simulink model "EPSAC_SM_BOOST"  (R2016a)
settings: Solver=VariableStepAuto  StartTime=0.0  StopTime=5  RelTol=1e-3
libraries: powerlib x11
settings Model: Creator=jorda  LastModifiedBy=jorda

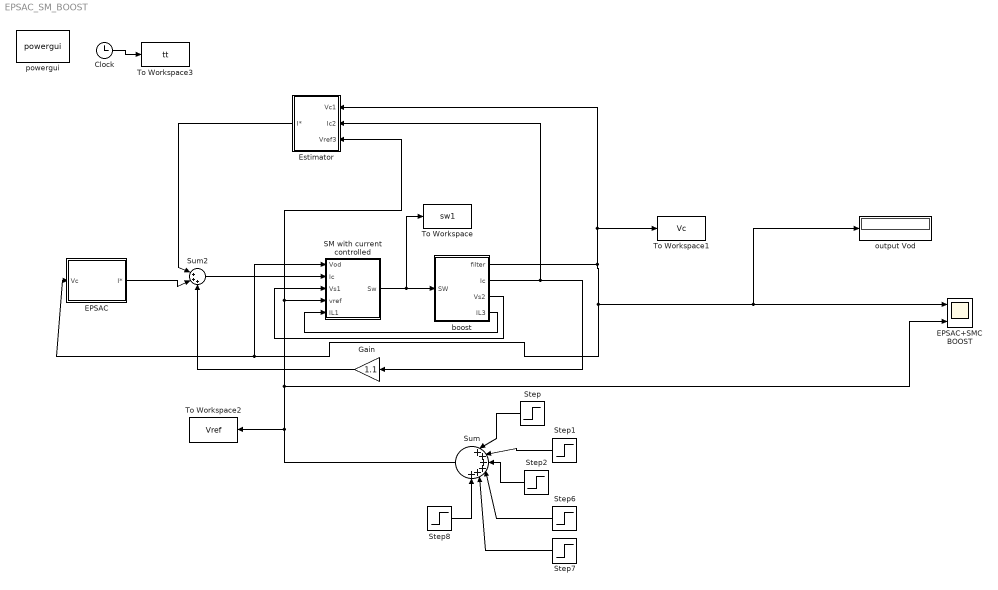
== system EPSAC_SM_BOOST ==
  Clock : Clock
  EPSAC : Subsystem
  EPSAC+SMC BOOST : Scope  NumInputPorts=2
  Estimator : Subsystem
  Gain : Gain  Gain=1.1
  SM with current controlled : Subsystem
  Step : Step  Time=0.5  Before=20  After=21  SampleTime=0
  Step1 : Step  SampleTime=0
  Step2 : Step  Time=1.5  After=-2  SampleTime=0
  Step6 : Step  Time=2  After=-1  SampleTime=0
  Step7 : Step  Time=2.5  After=-1  SampleTime=0
  Step8 : Step  Time=3  After=2  SampleTime=0
  Sum : Sum  Inputs=|++++++
  Sum2 : Sum  Inputs=|+++
  To Workspace : ToWorkspace  VariableName=sw1  SampleTime=1e-3
  To Workspace1 : ToWorkspace  VariableName=Vc  SampleTime=1e-3
  To Workspace2 : ToWorkspace  VariableName=Vref  SampleTime=1e-3
  To Workspace3 : ToWorkspace  VariableName=tt  SampleTime=1e-3
  boost : Subsystem
  output Vod : Display
  powergui : powerlib/powergui  Priority=1  SimulationMode=Continuous  SolverType=Tustin/Backward Euler (TBE)  SampleTime=50e-6  frequency=60  SPID=off  DisableSnubberDevices=off  DisableRonSwitches=off  DisableVfSwitches=off  SwTol=0  DisplayEquations=off  Interpol=off  ExternalGateDelay=off  methode=off  Ts=10  FunctionMessages=off  echomessages=off  HookPort=off  EnableUseOfTLC=off  x0status=blocks  frequencyindice=0  Pbase=100e6  ErrMax=1e-4  Iterations=50  UnitsV=kV  UnitsW=MW  buscounter=0  RestoreLinks=warning  ResistiveCurrentMeasurement=off  Frange=[0:2:500]  Ylog=off  Xlog=on  ShowGrid=off  save=off  variable=ZData  structure=0  ZoomFFT=off  StartTime=0.0  cycles=1  DisplayStyle=1  fundamental=60  FreqAxis=off  MaxFrequency=1000  frequencyindicesteady=1  RmsSteady=1  display=off
  wires:
  boost/3(Vs2) -> SM with current controlled/3("Vs1 ")
  boost/1(filter) -> output Vod/1, EPSAC+SMC BOOST/1, SM with current controlled/1(Vod), EPSAC/1(Vc), Estimator/1(Vc1), To Workspace1/1
  SM with current controlled/1(Sw) -> To Workspace/1, boost/1(SW)
  boost/2(Ic) -> Estimator/2(Ic2), Gain/1
  Clock/1 -> To Workspace3/1
  Gain/1 -> Sum2/3
  Step/1 -> Sum/1
  Step1/1 -> Sum/2
  Step2/1 -> Sum/3
  Step6/1 -> Sum/4
  Step7/1 -> Sum/5
  Step8/1 -> Sum/6
  Sum/1 -> To Workspace2/1, EPSAC+SMC BOOST/2, Estimator/3(Vref3), SM with current controlled/4(vref)
  boost/4(IL3) -> SM with current controlled/5(IL1)
  Sum2/1 -> SM with current controlled/2(Ic)
  EPSAC/1(I*) -> Sum2/2
  Estimator/1(I*) -> Sum2/1

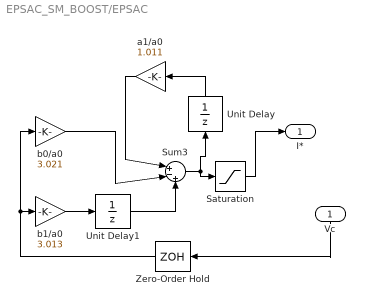
== system EPSAC_SM_BOOST/EPSAC ==
  Vc : Inport
  Saturation : Saturate  UpperLimit=0.4  LowerLimit=-0.4
  Sum3 : Sum  Inputs=|+-+
  Unit Delay : UnitDelay  SampleTime=1e-3
  Unit Delay1 : UnitDelay  SampleTime=1e-3
  Zero-Order Hold : ZeroOrderHold  SampleTime=1e-3
  a1/a0 : Gain  Gain=1.011
  b0/a0 : Gain  Gain=3.021
  b1/a0 : Gain  Gain=3.013
  I* : Outport
  wires:
  Vc/1 -> Zero-Order Hold/1
  Saturation/1 -> I*/1
  b0/a0/1 -> Sum3/2
  Zero-Order Hold/1 -> b0/a0/1, b1/a0/1
  b1/a0/1 -> Unit Delay1/1
  Unit Delay1/1 -> Sum3/3
  a1/a0/1 -> Sum3/1
  Unit Delay/1 -> a1/a0/1
  Sum3/1 -> Saturation/1, Unit Delay/1

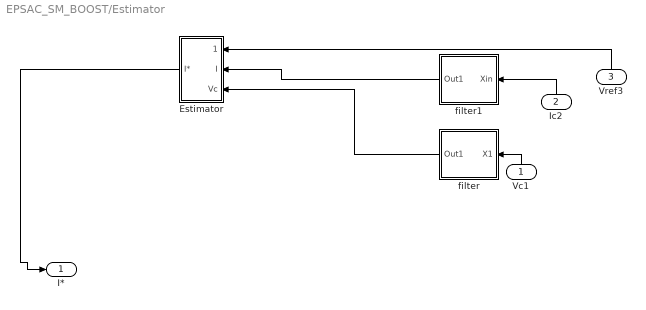
== system EPSAC_SM_BOOST/Estimator ==
  Vc1 : Inport
  Ic2 : Inport  Port=2
  Vref3 : Inport  Port=3
  Estimator : Subsystem
  filter : Subsystem
  filter1 : Subsystem
  I* : Outport
  wires:
  filter1/1(Out1) -> Estimator/2(I)
  Estimator/1(I*) -> I*/1
  Ic2/1 -> filter1/1(Xin)
  Vc1/1 -> filter/1(X1)
  Vref3/1 -> Estimator/1(Vref)
  filter/1(Out1) -> Estimator/3(Vc)

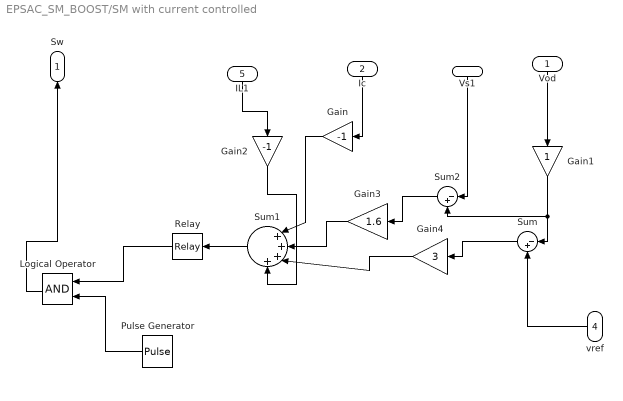
== system EPSAC_SM_BOOST/SM with current controlled ==
  Vod : Inport
  Ic : Inport  Port=2
  "Vs1 " : Inport  Port=3
  vref : Inport  Port=4
  IL1 : Inport  Port=5
  Gain : Gain  Gain=-1  ParamDataTypeStr=double  OutDataTypeStr=double
  Gain1 : Gain  ParamDataTypeStr=double  OutDataTypeStr=double
  Gain2 : Gain  Gain=-1  ParamDataTypeStr=double  OutDataTypeStr=double
  Gain3 : Gain  Gain=1.6  ParamDataTypeStr=double  OutDataTypeStr=double
  Gain4 : Gain  Gain=3  ParamDataTypeStr=double  OutDataTypeStr=double
  Logical Operator : Logic  AllPortsSameDT=off  OutDataTypeStr=boolean
  Pulse Generator : DiscretePulseGenerator  PulseType=Time based  Period=1e-3  PulseWidth=50
  Relay : Relay  OnSwitchValue=0.2  OffSwitchValue=-0.2  OutDataTypeStr=Inherit: Inherit via back propagation
  Sum : Sum  Inputs=|-+  AccumDataTypeStr=single  OutDataTypeStr=double  InputSameDT=on
  Sum1 : Sum  Inputs=|++++  AccumDataTypeStr=double  OutDataTypeStr=double  InputSameDT=on
  Sum2 : Sum  Inputs=|-+  AccumDataTypeStr=single  OutDataTypeStr=double  InputSameDT=on
  Sw : Outport
  wires:
  Gain1/1 -> Sum2/2, Sum/1
  "Vs1 "/1 -> Sum2/1
  Vod/1 -> Gain1/1
  Ic/1 -> Gain/1
  vref/1 -> Sum/2
  Sum/1 -> Gain4/1
  Sum2/1 -> Gain3/1
  Gain/1 -> Sum1/1
  Gain3/1 -> Sum1/2
  Gain4/1 -> Sum1/3
  Relay/1 -> Logical Operator/1
  Pulse Generator/1 -> Logical Operator/2
  Logical Operator/1 -> Sw/1
  Sum1/1 -> Relay/1
  IL1/1 -> Gain2/1
  Gain2/1 -> Sum1/4

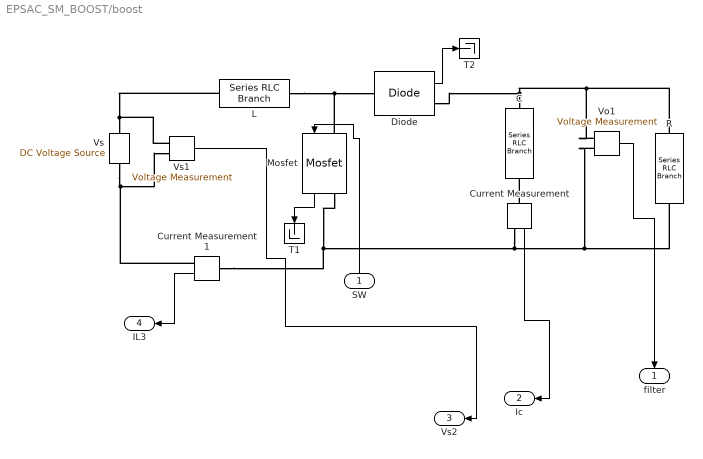
== system EPSAC_SM_BOOST/boost ==
  SW : Inport
  C : powerlib/Elements/Series RLC Branch  LConnTagsString=__new0  RConnTagsString=__new0  BranchType=C  Resistance=1  Inductance=1e-3  SetiL0=off  InitialCurrent=0  Capacitance=2000e-6  Setx0=off  InitialVoltage=0  Measurements=None
  Current Measurement : powerlib/Measurements/Current Measurement  PhasorSimulation=off  OutputType=Complex  PSBequivalent=0
  Current Measurement1 : powerlib/Measurements/Current Measurement  PhasorSimulation=off  OutputType=Complex  PSBequivalent=0
  Diode : powerlib/Power Electronics/Diode  Ron=0.001  Lon=0  Vf=0.8  IC=0  UseSnubber=off  Rs=500  Cs=250e-9  Measurements=on
  L : powerlib/Elements/Series RLC Branch  LConnTagsString=__new0  RConnTagsString=__new0  BranchType=L  Resistance=1  Inductance=2e-3  SetiL0=off  InitialCurrent=0  Capacitance=1e-6  Setx0=off  InitialVoltage=0  Measurements=None
  Mosfet : powerlib/Power Electronics/Mosfet  Ron=0.1  Lon=0  Rd=0.01  Vfd=0  IC=0  Rs=1e5  Cs=inf  Measurements=on
  R : powerlib/Elements/Series RLC Branch  LConnTagsString=__new0  RConnTagsString=__new0  BranchType=R  Resistance=4  Inductance=1e-3  SetiL0=off  InitialCurrent=0  Capacitance=1e-6  Setx0=off  InitialVoltage=0  Measurements=None
  T1 : Terminator
  T2 : Terminator
  Vo1 : powerlib/Measurements/Voltage Measurement  PhasorSimulation=off  OutputType=Complex  PSBequivalent=0
  Vs : powerlib/Electrical Sources/DC Voltage Source  Amplitude=15  Measurements=None
  Vs1 : powerlib/Measurements/Voltage Measurement  PhasorSimulation=off  OutputType=Complex  PSBequivalent=0
  filter : Outport
  Ic : Outport  Port=2
  Vs2 : Outport  Port=3
  IL3 : Outport  Port=4
  wires:
  Current Measurement/1 -> Ic/1
  Diode/1 -> T2/1
  Vs1/1 -> Vs2/1
  Mosfet/1 -> T1/1
  SW/1 -> Mosfet/1
  Vo1/1 -> filter/1
  Current Measurement1/1 -> IL3/1
  connections:
  Mosfet/LConn1 -- Diode/LConn1 -- L/RConn1
  L/LConn1 -- Vs1/LConn1 -- Vs/RConn1
  Mosfet/RConn1 -- Current Measurement1/LConn1 -- Current Measurement/RConn1 -- Vo1/LConn2 -- R/RConn1
  Vo1/LConn1 -- R/LConn1 -- Diode/RConn1 -- C/LConn1
  Current Measurement/LConn1 -- C/RConn1
  Vs/LConn1 -- Current Measurement1/RConn1 -- Vs1/LConn2

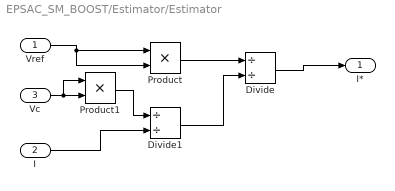
== system EPSAC_SM_BOOST/Estimator/Estimator ==
  Vref : Inport
  I : Inport  Port=2
  Vc : Inport  Port=3
  Divide : Product  Inputs=//
  Divide1 : Product  Inputs=//
  Product : Product
  Product1 : Product
  I* : Outport
  wires:
  Divide/1 -> I*/1
  Divide1/1 -> Divide/2
  Vref/1 -> Product/2, Product/1
  Product/1 -> Divide/1
  I/1 -> Divide1/2
  Vc/1 -> Product1/2, Product1/1
  Product1/1 -> Divide1/1

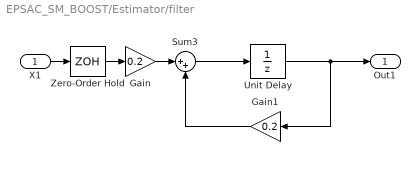
== system EPSAC_SM_BOOST/Estimator/filter ==
  X1 : Inport
  Gain : Gain  Gain=0.2
  Gain1 : Gain  Gain=0.2
  Sum3 : Sum  Inputs=|++
  Unit Delay : UnitDelay  SampleTime=1e-3
  Zero-Order Hold : ZeroOrderHold  SampleTime=1e-3
  Out1 : Outport
  wires:
  Unit Delay/1 -> Out1/1, Gain1/1
  Zero-Order Hold/1 -> Gain/1
  Sum3/1 -> Unit Delay/1
  X1/1 -> Zero-Order Hold/1
  Gain/1 -> Sum3/1
  Gain1/1 -> Sum3/2

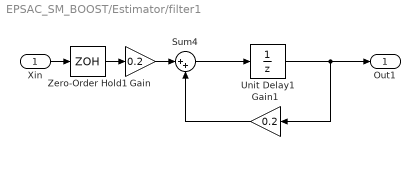
== system EPSAC_SM_BOOST/Estimator/filter1 ==
  Xin : Inport
  Gain : Gain  Gain=0.2
  Gain1 : Gain  Gain=0.2
  Sum4 : Sum  Inputs=|++
  Unit Delay1 : UnitDelay  SampleTime=1e-3
  Zero-Order Hold1 : ZeroOrderHold  SampleTime=1e-3
  Out1 : Outport
  wires:
  Unit Delay1/1 -> Out1/1, Gain1/1
  Zero-Order Hold1/1 -> Gain/1
  Sum4/1 -> Unit Delay1/1
  Xin/1 -> Zero-Order Hold1/1
  Gain/1 -> Sum4/1
  Gain1/1 -> Sum4/2
